simulink model "LQR_for_Nadir_Pointing"  (R2021a)
settings: Solver=FixedStepAuto  StartTime=0.0  StopTime=50  FixedStep=0.001  RelTol=1e-3
values from neighbouring files (symbols this model uses):
  B = inv(N)    [Para.m]    (also in Parameters.m = inv(N)*[zeros(3);eye(3)])
  N = [eye(3) zeros(3);zeros(3) J]    [Dynamics.m]    (also in Para.m; Parameters.m)
  R = eye(6)    [Para.m]    (also in Parameters.m = eye(3))
  S = [0 0 0 0.5 0 0;           0 0 0 0 0.5 0;           0 0 0 0 0 0.5;           f41 0 0 0 0 f46;           0 f52 0 0 0 0;           0 0 f63 f64 0 0]    [Para.m]    (also in Parameters.m; crossMatrix.m = [0 -q3 q2;           q3 0 -q1;           -q2 q1 0])
undefined symbols (not defined in the file or in its folder): F
settings Model: Creator=VTX  LastModifiedBy=VTX

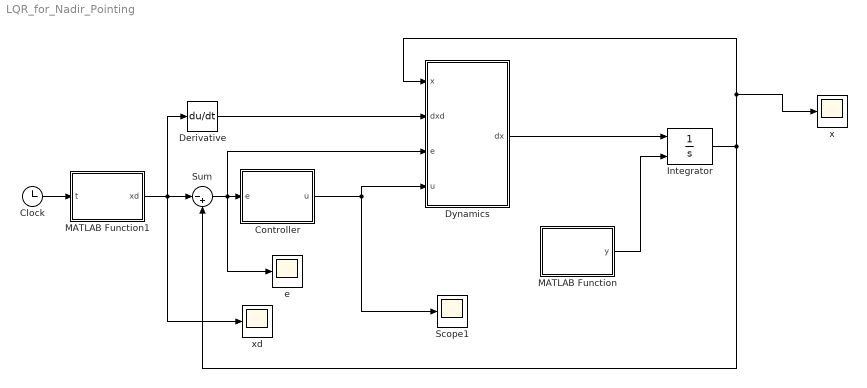
== system LQR_for_Nadir_Pointing ==
  Clock : Clock
  Controller : MATLAB Function  TreatAsAtomicUnit=on
  Derivative : Derivative
  Dynamics : MATLAB Function  TreatAsAtomicUnit=on
  Integrator : Integrator  InitialConditionSource=external
  MATLAB Function : MATLAB Function  TreatAsAtomicUnit=on
  MATLAB Function1 : MATLAB Function  TreatAsAtomicUnit=on
  Scope1 : Scope
  Sum : Sum  Inputs=|-+
  e : Scope
  x : Scope
  xd : Scope
  wires:
  Controller/1(u) -> Dynamics/4(u), Scope1/1
  Dynamics/1(dx) -> Integrator/1
  Integrator/1 -> Sum/2, Dynamics/1(x), x/1
  MATLAB Function/1(y) -> Integrator/2
  Sum/1 -> e/1, Dynamics/3(e), Controller/1(e)
  MATLAB Function1/1(xd) -> xd/1, Derivative/1, Sum/1
  Derivative/1 -> Dynamics/2(dxd)
  Clock/1 -> MATLAB Function1/1(t)

== matlab function LQR_for_Nadir_Pointing/Controller ==
  data: e input; u output; F parameter; B parameter; R parameter
function u = fcn(e, F, B, R)
%% Controller
   u = -inv(R)*B'*F*e;
end

== matlab function LQR_for_Nadir_Pointing/Dynamics ==
  data: x input; dxd input; e input; dx output; u input; N parameter; S parameter
function dx  = fcn(x,dxd,e,u,N,S)
%% Quaternions
    %q = [q1 q2 q3]';
    %quater = [q0 q']';
    q = x(1:3,:);
    
%% Angular velocity
    omega_BR = x(4:6,:);
    
%% State Model: dx = Ax + Bu
    %dx = inv(N)*(S*[q' omega_BR']' + [0 0 0 u']');
    dx = dxd + inv(N)*(S*e + [0 0 0 u']');
    dq = dx(1:3,:);
    domega = dx(4:6,:);
end

== matlab function LQR_for_Nadir_Pointing/MATLAB Function ==
  data: y output
function y = fcn()
    y = rand(6,1);
end

== matlab function LQR_for_Nadir_Pointing/MATLAB Function1 ==
  data: t input; xd output
function xd = fcn(t)
    xd = [sin(0.5*t) cos(0.25*t) 5*sin(0.25*t) (sin(t)+sin(0.5*t)) 2*cos(t) cos(t)]';
end
